simulink model "Summation_odd"  (R2019b)
settings: Solver=FixedStepAuto  StartTime=0.0  StopTime=3  FixedStep=1  RelTol=1e-3
libraries: simulink x1
settings Model: Creator=Rashedul Islam  LastModifiedBy=Rashedul Islam

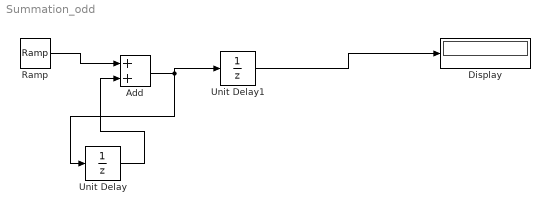
== system Summation_odd ==
  Add : Sum
  Display : Display
  Ramp : simulink/Sources/Ramp  slope=2  start=0  InitialOutput=1
  Unit Delay : UnitDelay  SampleTime=-1  HasFrameUpgradeWarning=on
  Unit Delay1 : UnitDelay  SampleTime=-1  HasFrameUpgradeWarning=on
  wires:
  Add/1 -> Unit Delay1/1, Unit Delay/1
  Unit Delay/1 -> Add/2
  Ramp/1 -> Add/1
  Unit Delay1/1 -> Display/1
